simulink model "thermal_model"  (R2023b)
settings: Solver=VariableStepAuto  StartTime=0.0  StopTime=240  RelTol=1e-3
undefined symbols (not defined in the file or in its folder): C_HA, C_WA, R_HA, R_WA, R_WH
settings Model: Creator=rgpieper  LastModifiedBy=rgpieper
settings ModelReferenceCC: EnableRefExpFcnMdlSchedulingChecks=on

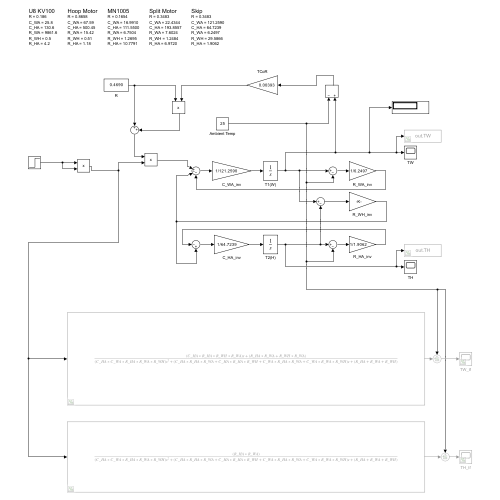
[thumbnail: Simulink's stored preview of the top-level diagram]
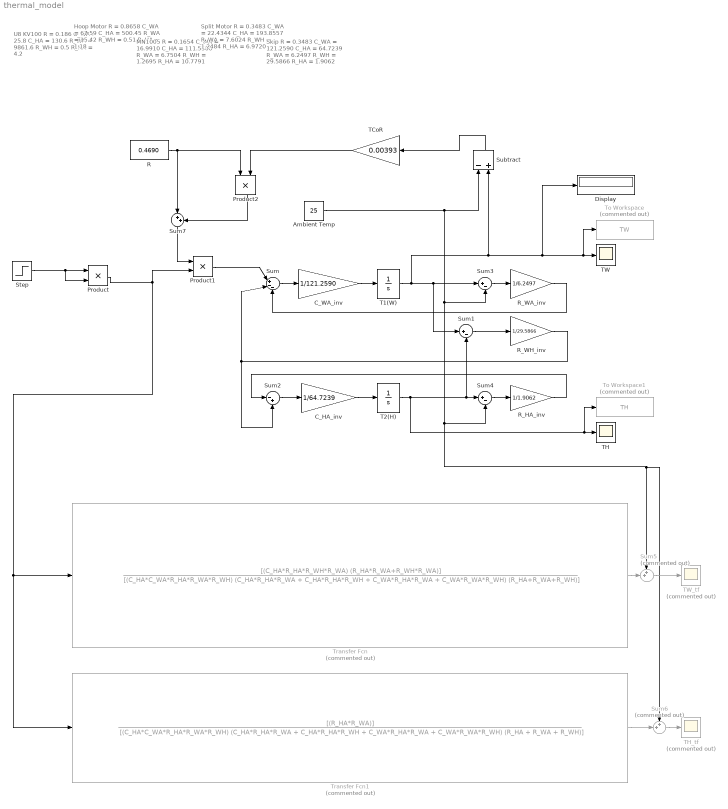
== system thermal_model ==
  note: U8 KV100
      | R = 0.186
      | C_WA = 25.8
      | C_HA = 130.6
      | R_WA = 9861.6
      | R_WH = 0.5
      | R_HA = 4.2
  note: Hoop Motor
      | R = 0.8658
      | C_WA = 67.59
      | C_HA = 500.45
      | R_WA = 15.42
      | R_WH = 0.51
      | R_HA = 1.18
  note: MN1005
      | R = 0.1654
      | C_WA = 16.9910
      | C_HA = 111.5500
      | R_WA = 6.7504
      | R_WH = 1.2695
      | R_HA = 10.7791
  note: Split Motor
      | R = 0.3483
      | C_WA = 22.4344
      | C_HA = 193.8557
      | R_WA = 7.6024
      | R_WH = 1.2484
      | R_HA = 6.9720
  note: Skip
      | R = 0.3483
      | C_WA = 121.2590
      | C_HA = 64.7239
      | R_WA = 6.2497
      | R_WH = 29.5866
      | R_HA = 1.9062
  Ambient Temp : Constant  Value=25
  C_HA_inv : Gain  Gain=1/64.7239
  C_WA_inv : Gain  Gain=1/121.2590
  Display : Display
  Product : Product
  Product1 : Product
  Product2 : Product
  R : Constant  Value=0.4690
  R_HA_inv : Gain  Gain=1/1.9062
  R_WA_inv : Gain  Gain=1/6.2497
  R_WH_inv : Gain  Gain=1/29.5866
  Step : Step  Time=0  After=10  SampleTime=0
  Subtract : Sum  Inputs=-+
  Sum : Sum  Inputs=|+--
  Sum1 : Sum  Inputs=|+-
  Sum2 : Sum  Inputs=|-+
  Sum3 : Sum  Inputs=|+-
  Sum4 : Sum  Inputs=|+-
  Sum5 : Sum  Commented=on  Inputs=++|
  Sum6 : Sum  Commented=on  Inputs=++|
  Sum7 : Sum  Inputs=|++
  T1(W) : Integrator  InitialCondition=25  ContinuousStateAttributes="\"T1\""
  T2(H) : Integrator  InitialCondition=25  ContinuousStateAttributes='T2'
  TCoR : Gain  Gain=0.00393
  TH : Scope
  TH_tf : Scope  Commented=on
  TW : Scope
  TW_tf : Scope  Commented=on
  To Workspace : ToWorkspace  Commented=on  VariableName=TW  SaveFormat=Timeseries  SampleTime=1
  To Workspace1 : ToWorkspace  Commented=on  VariableName=TH  SaveFormat=Timeseries  SampleTime=1
  Transfer Fcn : TransferFcn  Commented=on  Numerator=[(C_HA*R_HA*R_WH*R_WA) (R_HA*R_WA+R_WH*R_WA)]  Denominator=[(C_HA*C_WA*R_HA*R_WA*R_WH) (C_HA*R_HA*R_WA + C_HA*R_HA*R_WH + C_WA*R_HA*R_WA + C_WA*R_WA*R_WH) (R_HA+R_WA+R_WH)]
  Transfer Fcn1 : TransferFcn  Commented=on  Numerator=[(R_HA*R_WA)]  Denominator=[(C_HA*C_WA*R_HA*R_WA*R_WH) (C_HA*R_HA*R_WA + C_HA*R_HA*R_WH + C_WA*R_HA*R_WA + C_WA*R_WA*R_WH) (R_HA + R_WA + R_WH)]
  wires:
  Step/1 -> Product/2, Product/1
  Product/1 -> Transfer Fcn1/1, Transfer Fcn/1, Product1/2
  Product1/1 -> Sum/1
  Sum/1 -> C_WA_inv/1
  C_WA_inv/1 -> T1(W)/1
  C_HA_inv/1 -> T2(H)/1
  T2(H)/1 -> Sum1/2, Sum4/1, To Workspace1/1, TH/1
  Sum1/1 -> R_WH_inv/1
  R_WH_inv/1 -> Sum/2, Sum2/2
  Sum2/1 -> C_HA_inv/1
  Sum3/1 -> R_WA_inv/1
  Ambient Temp/1 -> Subtract/1, Sum6/1, Sum5/1, Sum4/2, Sum3/2
  R_WA_inv/1 -> Sum/3
  Sum4/1 -> R_HA_inv/1
  R_HA_inv/1 -> Sum2/1
  T1(W)/1 -> Display/1, To Workspace/1, TW/1, Subtract/2, Sum3/1, Sum1/1
  Transfer Fcn/1 -> Sum5/2
  Sum5/1 -> TW_tf/1
  Sum6/1 -> TH_tf/1
  Transfer Fcn1/1 -> Sum6/2
  Subtract/1 -> TCoR/1
  TCoR/1 -> Product2/2
  R/1 -> Product2/1, Sum7/1
  Product2/1 -> Sum7/2
  Sum7/1 -> Product1/1
